simulink model "VCU_SW"  (R2020b)
settings: Solver=FixedStepDiscrete  StartTime=0.0  StopTime=inf  FixedStep=1e-2  RelTol=1e-3
PreLoadFcn:
  | RTWConfigurationCB('preloadfcn', bdroot);
InitFcn:
  | loadvar_ttc500
undefined symbols (not defined in the file or in its folder): BrkPedalTypes, CabMovModeTypes, cFuseTempSensAcc_X, cFuseTempSensAcc_Y, cFuseTempSensVal_X, cFuseTempSensVal_Y, cTMSTempSensVal_X, cTMSTempSensVal_Y, cTransferCaseSpeedRatio, diag_state, DoorsPositionTypes, dP_filter_Y, DriverOccClassSystemTypes, ErrorValueTypes, fatal_error_callback, IO_ADC_NO_RANGE, LadderStatusTypes, pAnalogCabRotSensAcc, pAnalogCabRotSensMaxVolt, pAnalogCabRotSensMinVolt, pAnalogCabRotSensRange, pAnalogCabRotSensZeroVolt, pBrkActivePress, pCabTiltSensAcc, pCabTiltSensMaxCur, pCabTiltSensMinCur, pDistanceCorrection, pECANManual_BPNEnable, pECANManual_BPNEnabler_Flag, pFilterSensAccRes, pHDirMaxDiffFrq, pHDirSensHighLvl, pHDirSensLowLvl, pMainGearRatio, pMaxFilterSensRes, pMaxFirstPedalSensValue, pMaxFuseTempSensRes, pMaxPressLoss, pMaxPressSensCurrent, pMaxPressValue, pMaxPressValueHydMotAndPump, pMaxPressValueParkDrain, pMaxSecondPedalSensValue, pMaxTempSensVoltage, pMaxTempValue, pMaxTMSTempSensRes, pMinFilterSensRes, pMinFirstPedalSensValue, pMinFuseTempSensRes, pMinPressLoss, pMinPressSensCurrent, pMinPressValue, pMinSecondPedalSensValue, pMinTempSensVoltage, pMinTempValue, pMinTMSTempSensRes, pMotorRingTeethNum, pPedalSensAccuracyPct, pPedalSensAccuracyVolt, pPressLossTreshhold ... (+20)
libraries: TTlibrary x271, canmsglib x128, simulink x88
(part 13 of 17)

== system VCU_SW/OutputLayer/OutputNetwork/OutputCCAN/SetCCAN1000msec/Eletcric_current_info ==
  CANPack_Electric_current_info : canmsglib/CAN Pack  MsgList=(none)  MsgName=Electric_current_info  MsgIDType=Extended (29-bit identifier)  MsgIdentifier=419386874  MsgLength=8  Remote=off  ApplyMinMax=off  BusOutput=on  SignalInfo={ 'equp_pump_cur', '48', '16', 'LE', 'unsigned', 'Standard', '0', '1', '0', '0', '65535'; 'front_drive_hydpump_cur', '0', '16', 'LE', 'unsigned', 'Standard', '0', '1', '0', '0', '65535'; 'hydmot_cur', '32', '16', 'LE', 'unsigned', 'Standard', '0', '1', '0', '0', '65535'; 'reverse_drive_hydpump_cur', '16', '16', 'LE', 'unsigned', 'Standard', '0', '1', '0', '0', '65535' }
      settings: SourceProductBaseCode=ME,XP,VN  DataFormat=manually specified signals
  Data Store Read : DataStoreRead  DataStoreName=OutputNetworkData  DataStoreElements=OutputNetworkData.CCAN.Electric_current_info.equp_pump_cur#OutputNetworkData.CCAN.Electric_current_info.front_drive_hydpump_cur#OutputNetworkData.CCAN.Electric_current_info.hydmot_cur#OutputNetworkData.CCAN.Electric_current_info.reverse_drive_hydpump_cur
  Terminator1 : Terminator
  transmit_message_electric_current_info : TTlibrary/CAN/transmit_message_name  channel=IO_CAN_CHANNEL_1  id_format=IO_CAN_STD_FRAME  retranslation=off  io_error=on  sample_time=-1
      settings: SourceProductName=TT control 500 series
  wires:
  transmit_message_electric_current_info/1 -> Terminator1/1  "error_tx_transmit_message_electric_current_info"
  CANPack_Electric_current_info/1 -> transmit_message_electric_current_info/1
  Data Store Read/1 -> CANPack_Electric_current_info/1
  Data Store Read/2 -> CANPack_Electric_current_info/2
  Data Store Read/3 -> CANPack_Electric_current_info/3
  Data Store Read/4 -> CANPack_Electric_current_info/4

== system VCU_SW/OutputLayer/OutputNetwork/OutputCCAN/SetCCAN1000msec/Eletcric_info ==
  CANPack_Electric_info : canmsglib/CAN Pack  MsgList=(none)  MsgName=Electric_info  MsgIDType=Extended (29-bit identifier)  MsgIdentifier=419387130  MsgLength=8  Remote=off  ApplyMinMax=off  BusOutput=on  SignalInfo={ 'bort_batt_voltage_lvl', '0', '8', 'LE', 'unsigned', 'Standard', '0', '1', '0', '0', '255'; 'can1_sts', '32', '2', 'LE', 'unsigned', 'Standard', '0', '1', '0', '0', '3'; 'can2_sts', '34', '2', 'LE', 'unsigned', 'Standard', '0', '1', '0', '0', '3'; 'can3_sts', '36', '2', 'LE', 'unsigned', 'Standard', '0', '1', '0', '0', '3'; 'can4_sts', '38', '2', 'LE', 'unsigned', 'Standard', '0', '1', '0', '0', '3'; 'can5_sts', '40', '2', 'LE', 'unsigned', 'Standard', '0', '1', '0', '0', '3'; 'can6_sts', '42', '2', 'LE', 'unsigned', 'Standard', '0', '1', '0', '0', '3'; 'lower_gen_signal', '10', '2', 'LE', 'unsigned', 'Standard', '0', '1', '0', '0', '3'; 'str_brk_pump_cur', '16', '16', 'LE', 'unsigned', 'Standard', '0', '1', '0', '0', '65535'; 'upper_gen_signal', '8', '2', 'LE', 'unsigned', 'Standard', '0', '1', '0', '0', '3' }
      settings: SourceProductBaseCode=ME,XP,VN  DataFormat=manually specified signals
  Data Store Read : DataStoreRead  DataStoreName=OutputNetworkData  DataStoreElements=OutputNetworkData.CCAN.Electric_info.bort_batt_voltage_lvl#OutputNetworkData.CCAN.Electric_info.can1_sts#OutputNetworkData.CCAN.Electric_info.can2_sts#OutputNetworkData.CCAN.Electric_info.can3_sts#OutputNetworkData.CCAN.Electric_info.can4_sts#OutputNetworkData.CCAN.Electric_info.can5_sts#OutputNetworkData.CCAN.Electric_info.can6_sts#OutputNetworkData.CCAN.Electric_info.lower_gen_signal#OutputNetworkData.CCAN.Electric_info.str_brk_pump_cur#OutputNetworkData.CCAN.Electric_info.bort_batt_voltage_lvl
  Terminator1 : Terminator
  transmit_message_electric_info : TTlibrary/CAN/transmit_message_name  channel=IO_CAN_CHANNEL_1  id_format=IO_CAN_STD_FRAME  retranslation=off  io_error=on  sample_time=-1
      settings: SourceProductName=TT control 500 series
  wires:
  CANPack_Electric_info/1 -> transmit_message_electric_info/1
  transmit_message_electric_info/1 -> Terminator1/1  "error_tx_transmit_message_electric_info"
  Data Store Read/1 -> CANPack_Electric_info/1
  Data Store Read/2 -> CANPack_Electric_info/2
  Data Store Read/3 -> CANPack_Electric_info/3
  Data Store Read/4 -> CANPack_Electric_info/4
  Data Store Read/5 -> CANPack_Electric_info/5
  Data Store Read/6 -> CANPack_Electric_info/6
  Data Store Read/7 -> CANPack_Electric_info/7
  Data Store Read/8 -> CANPack_Electric_info/8
  Data Store Read/9 -> CANPack_Electric_info/9
  Data Store Read/10 -> CANPack_Electric_info/10

== system VCU_SW/OutputLayer/OutputNetwork/OutputCCAN/SetCCAN1000msec/HTR ==
  CANPack_HTR : canmsglib/CAN Pack  MsgList=(none)  MsgName=HTR  MsgIDType=Extended (29-bit identifier)  MsgIdentifier=419327482  MsgLength=8  Remote=off  ApplyMinMax=off  BusOutput=on  SignalInfo={ 'AuxiliaryHeaterMode', '24', '4', 'LE', 'unsigned', 'Standard', '0', '1', '0', '0', '15' }
      settings: SourceProductBaseCode=ME,XP,VN  DataFormat=manually specified signals
  Data Store Read1 : DataStoreRead  DataStoreName=OutputNetworkData  DataStoreElements=OutputNetworkData.CCAN.HTR.AuxiliaryHeaterMode
  Terminator1 : Terminator
  transmit_message_htr : TTlibrary/CAN/transmit_message_name  channel=IO_CAN_CHANNEL_1  id_format=IO_CAN_STD_FRAME  retranslation=off  io_error=on  sample_time=-1
      settings: SourceProductName=TT control 500 series
  wires:
  CANPack_HTR/1 -> transmit_message_htr/1
  Data Store Read1/1 -> CANPack_HTR/1
  transmit_message_htr/1 -> Terminator1/1  "error_tx_transmit_message_htr"

== system VCU_SW/OutputLayer/OutputNetwork/OutputCCAN/SetCCAN1000msec/Hyd_transm_info ==
  CANPack_Hyd_transm_info : canmsglib/CAN Pack  MsgList=(none)  MsgName=Hyd_transm_info  MsgIDType=Extended (29-bit identifier)  MsgIdentifier=419386362  MsgLength=8  Remote=off  ApplyMinMax=off  BusOutput=on  SignalInfo={ 'front_drive_line_press', '0', '8', 'LE', 'unsigned', 'Standard', '0', '2', '0', '0', '510'; 'hyd_mot_temp_sens', '16', '8', 'LE', 'unsigned', 'Standard', '0', '1', '-40', '-40', '210'; 'hyd_pump_temp_sens', '24', '8', 'LE', 'unsigned', 'Standard', '0', '1', '-40', '-40', '210'; 'hydmot_direct_sens', '40', '2', 'LE', 'unsigned', 'Standard', '0', '1', '0', '0', '3'; 'hydpump_direct_sens', '48', '2', 'LE', 'unsigned', 'Standard', '0', '1', '0', '0', '3'; 'hydpump_washer_lean_sens', '32', '8', 'LE', 'unsigned', 'Standard', '0', '1', '0', '0', '255'; 'rear_drive_line_press', '8', '8', 'LE', 'unsigned', 'Standard', '0', '2', '0', '0', '510' }
      settings: SourceProductBaseCode=ME,XP,VN  DataFormat=manually specified signals
  Data Store Read : DataStoreRead  DataStoreName=OutputNetworkData  DataStoreElements=OutputNetworkData.CCAN.Hyd_transm_info.front_drive_line_press#OutputNetworkData.CCAN.Hyd_transm_info.hyd_mot_temp_sens#OutputNetworkData.CCAN.Hyd_transm_info.hyd_pump_temp_sens#OutputNetworkData.CCAN.Hyd_transm_info.hydmot_direct_sens#OutputNetworkData.CCAN.Hyd_transm_info.hydpump_direct_sens#OutputNetworkData.CCAN.Hyd_transm_info.hydpump_washer_lean_sens#OutputNetworkData.CCAN.Hyd_transm_info.rear_drive__line_press
  Terminator1 : Terminator
  transmit_message_hyd_transm_info : TTlibrary/CAN/transmit_message_name  channel=IO_CAN_CHANNEL_1  id_format=IO_CAN_STD_FRAME  retranslation=off  io_error=on  sample_time=-1
      settings: SourceProductName=TT control 500 series
  wires:
  transmit_message_hyd_transm_info/1 -> Terminator1/1  "error_tx_transmit_message_hyd_transm_info"
  CANPack_Hyd_transm_info/1 -> transmit_message_hyd_transm_info/1
  Data Store Read/1 -> CANPack_Hyd_transm_info/1
  Data Store Read/2 -> CANPack_Hyd_transm_info/2
  Data Store Read/3 -> CANPack_Hyd_transm_info/3
  Data Store Read/4 -> CANPack_Hyd_transm_info/4
  Data Store Read/5 -> CANPack_Hyd_transm_info/5
  Data Store Read/6 -> CANPack_Hyd_transm_info/6
  Data Store Read/7 -> CANPack_Hyd_transm_info/7

== system VCU_SW/OutputLayer/OutputNetwork/OutputCCAN/SetCCAN1000msec/Hyd_transm_speed_info ==
  CANPack_Hyd_transm_speed_info : canmsglib/CAN Pack  MsgList=(none)  MsgName=Hyd_transm_speed_info  MsgIDType=Extended (29-bit identifier)  MsgIdentifier=419386618  MsgLength=8  Remote=off  ApplyMinMax=off  BusOutput=on  SignalInfo={ 'hydmot_speed_sens_1', '32', '16', 'LE', 'unsigned', 'Standard', '0', '0.125', '0', '0', '8191.88'; 'hydmot_speed_sens_2', '48', '16', 'LE', 'unsigned', 'Standard', '0', '0.125', '0', '0', '8191.88'; 'hydpump_speed_sens_1', '0', '16', 'LE', 'unsigned', 'Standard', '0', '0.125', '0', '0', '8191.875'; 'hydpump_speed_sens_2', '16', '16', 'LE', 'unsigned', 'Standard', '0', '0.125', '0', '0', '8191.875' }
      settings: SourceProductBaseCode=ME,XP,VN  DataFormat=manually specified signals
  Data Store Read : DataStoreRead  DataStoreName=OutputNetworkData  DataStoreElements=OutputNetworkData.CCAN.Hyd_transm_speed_info.hydmot_speed_sens_1#OutputNetworkData.CCAN.Hyd_transm_speed_info.hydmot_speed_sens_2#OutputNetworkData.CCAN.Hyd_transm_speed_info.hydpump_speed_sens_1#OutputNetworkData.CCAN.Hyd_transm_speed_info.hydpump_speed_sens_2
  Data Type Conversion{,1..3} (4 alike) : DataTypeConversion  OutDataTypeStr=single
  Terminator1 : Terminator
  transmit_message_hyd_transm_speed_info : TTlibrary/CAN/transmit_message_name  channel=IO_CAN_CHANNEL_1  id_format=IO_CAN_STD_FRAME  retranslation=off  io_error=on  sample_time=-1
      settings: SourceProductName=TT control 500 series
  wires:
  CANPack_Hyd_transm_speed_info/1 -> transmit_message_hyd_transm_speed_info/1
  transmit_message_hyd_transm_speed_info/1 -> Terminator1/1  "error_tx_transmit_message_hyd_transm_speed_info"
  Data Store Read/1 -> Data Type Conversion/1
  Data Store Read/2 -> Data Type Conversion1/1
  Data Store Read/3 -> Data Type Conversion2/1
  Data Store Read/4 -> Data Type Conversion3/1
  Data Type Conversion/1 -> CANPack_Hyd_transm_speed_info/1
  Data Type Conversion1/1 -> CANPack_Hyd_transm_speed_info/2
  Data Type Conversion2/1 -> CANPack_Hyd_transm_speed_info/3
  Data Type Conversion3/1 -> CANPack_Hyd_transm_speed_info/4

== system VCU_SW/OutputLayer/OutputNetwork/OutputCCAN/SetCCAN1000msec/LCMD ==
  CANPack_LCMD_VCU : canmsglib/CAN Pack  MsgList=(none)  MsgName=LCMD_VCU  MsgIDType=Extended (29-bit identifier)  MsgIdentifier=217989626  MsgLength=3  Remote=off  ApplyMinMax=off  BusOutput=on  SignalInfo={ 'CenterStopLightCmd', '18', '2', 'LE', 'unsigned', 'Standard', '0', '1', '0', '0', '3'; 'LeftStopLightCmd', '22', '2', 'LE', 'unsigned', 'Standard', '0', '1', '0', '0', '3'; 'RightStopLightCmd', '20', '2', 'LE', 'unsigned', 'Standard', '0', '1', '0', '0', '3' }
      settings: SourceProductBaseCode=ME,XP,VN  DataFormat=manually specified signals
  Data Store Read1 : DataStoreRead  DataStoreName=OutputNetworkData  DataStoreElements=OutputNetworkData.CCAN.LD_out.CenterStopLight#OutputNetworkData.CCAN.LD_out.LeftStopLight#OutputNetworkData.CCAN.LD_out.RightStopLight
  Terminator1 : Terminator
  transmit_message_lcmd_vcu : TTlibrary/CAN/transmit_message_name  channel=IO_CAN_CHANNEL_1  id_format=IO_CAN_STD_FRAME  retranslation=off  io_error=on  sample_time=-1
      settings: SourceProductName=TT control 500 series
  wires:
  Data Store Read1/3 -> CANPack_LCMD_VCU/3
  Data Store Read1/2 -> CANPack_LCMD_VCU/2
  Data Store Read1/1 -> CANPack_LCMD_VCU/1
  transmit_message_lcmd_vcu/1 -> Terminator1/1  "error_tx_transmit_message_lcmd_vcu"
  CANPack_LCMD_VCU/1 -> transmit_message_lcmd_vcu/1

== system VCU_SW/OutputLayer/OutputNetwork/OutputCCAN/SetCCAN1000msec/MTUInformationArea ==
  CANPack_MTUInformationArea : canmsglib/CAN Pack  MsgList=(none)  MsgName=MTUInformationArea  MsgIDType=Extended (29-bit identifier)  MsgIdentifier=419386106  MsgLength=8  Remote=off  ApplyMinMax=off  BusOutput=on  SignalInfo={ 'info_area_id', '0', '8', 'LE', 'unsigned', 'Standard', '0', '1', '0', '0', '255' }
      settings: SourceProductBaseCode=ME,XP,VN  DataFormat=manually specified signals
  Ground : Ground
  Terminator1 : Terminator
  transmit_message_mtu_information_area : TTlibrary/CAN/transmit_message_name  channel=IO_CAN_CHANNEL_1  id_format=IO_CAN_STD_FRAME  retranslation=off  io_error=on  sample_time=-1
      settings: SourceProductName=TT control 500 series
  wires:
  CANPack_MTUInformationArea/1 -> transmit_message_mtu_information_area/1
  Ground/1 -> CANPack_MTUInformationArea/1
  transmit_message_mtu_information_area/1 -> Terminator1/1  "error_tx_transmit_message_mtu_information_area"

== system VCU_SW/OutputLayer/OutputNetwork/OutputCCAN/SetCCAN1000msec/TCI ==
  CANPack_TCI : canmsglib/CAN Pack  MsgList=(none)  MsgName=TCI  MsgIDType=Extended (29-bit identifier)  MsgIdentifier=419267578  MsgLength=8  Remote=off  ApplyMinMax=off  BusOutput=on  SignalInfo={ 'Transfer_Case_Status', '0', '3', 'LE', 'unsigned', 'Standard', '0', '1', '0', '0', '7' }
      settings: SourceProductBaseCode=ME,XP,VN  DataFormat=manually specified signals
  Data Store Read1 : DataStoreRead  DataStoreName=OutputNetworkData  DataStoreElements=OutputNetworkData.CCAN.TCI.Transfer_Case_Status
  Terminator1 : Terminator
  transmit_message_tci : TTlibrary/CAN/transmit_message_name  channel=IO_CAN_CHANNEL_1  id_format=IO_CAN_STD_FRAME  retranslation=off  io_error=on  sample_time=-1
      settings: SourceProductName=TT control 500 series
  wires:
  transmit_message_tci/1 -> Terminator1/1  "error_tx_transmit_message_tci"
  Data Store Read1/1 -> CANPack_TCI/1
  CANPack_TCI/1 -> transmit_message_tci/1

== system VCU_SW/OutputLayer/OutputNetwork/OutputCCAN/SetCCAN1000msec/TRF2 ==
  CANPack_TRF2 : canmsglib/CAN Pack  MsgList=(none)  MsgName=TRF2  MsgIDType=Extended (29-bit identifier)  MsgIdentifier=419272186  MsgLength=8  Remote=off  ApplyMinMax=off  BusOutput=on  SignalInfo={ 'Transmission_Overheat_Indicator', '4', '2', 'LE', 'unsigned', 'Standard', '0', '1', '0', '0', '3' }
      settings: SourceProductBaseCode=ME,XP,VN  DataFormat=manually specified signals
  Data Store Read1 : DataStoreRead  DataStoreName=OutputNetworkData  DataStoreElements=OutputNetworkData.CCAN.TRF2.Transmission_Overheat_Indicator
  Terminator1 : Terminator
  transmit_message_trf2 : TTlibrary/CAN/transmit_message_name  channel=IO_CAN_CHANNEL_1  id_format=IO_CAN_STD_FRAME  retranslation=off  io_error=on  sample_time=-1
      settings: SourceProductName=TT control 500 series
  wires:
  CANPack_TRF2/1 -> transmit_message_trf2/1
  Data Store Read1/1 -> CANPack_TRF2/1
  transmit_message_trf2/1 -> Terminator1/1  "error_tx_transmit_message_trf2"

== system VCU_SW/OutputLayer/OutputNetwork/OutputCCAN/SetCCAN1000msec/VH ==
  CANPack_VH : canmsglib/CAN Pack  MsgList=(none)  MsgName=VH  MsgIDType=Extended (29-bit identifier)  MsgIdentifier=419358714  MsgLength=8  Remote=off  ApplyMinMax=off  BusOutput=on  SignalInfo={ 'TotalVehicleHours', '0', '32', 'LE', 'unsigned', 'Standard', '0', '0.05', '0', '0', '210554060.75'; 'TripVehicleHours', '32', '32', 'LE', 'unsigned', 'Standard', '0', '0.05', '0', '0', '210554000' }
      settings: SourceProductBaseCode=ME,XP,VN  DataFormat=manually specified signals
  Data Store Read1 : DataStoreRead  DataStoreName=OutputNetworkData  DataStoreElements=OutputNetworkData.CCAN.VH.TotalVehicleHours
  Data Store Read2 : DataStoreRead  DataStoreName=OutputNetworkData  DataStoreElements=OutputNetworkData.CCAN.VH.TripVehicleHours
  Terminator1 : Terminator
  transmit_message_vh : TTlibrary/CAN/transmit_message_name  channel=IO_CAN_CHANNEL_1  id_format=IO_CAN_STD_FRAME  retranslation=off  io_error=on  sample_time=-1
      settings: SourceProductName=TT control 500 series
  wires:
  CANPack_VH/1 -> transmit_message_vh/1
  Data Store Read1/1 -> CANPack_VH/1
  transmit_message_vh/1 -> Terminator1/1  "error_tx_transmit_message_vh"
  Data Store Read2/1 -> CANPack_VH/2

== system VCU_SW/OutputLayer/OutputNetwork/OutputCCAN/SetCCAN100msec/CCVS1 ==
  CANPack_CCVS1 : canmsglib/CAN Pack  MsgList=(none)  MsgName=CCVS1  MsgIDType=Extended (29-bit identifier)  MsgIdentifier=419361274  MsgLength=8  Remote=off  ApplyMinMax=off  BusOutput=on  SignalInfo={ 'Brake_Switch', '28', '2', 'LE', 'unsigned', 'Standard', '0', '1', '0', '0', '3'; 'PTO_Governor_State', '48', '5', 'LE', 'unsigned', 'Standard', '0', '1', '0', '0', '32'; 'Parking_Brake_Switch', '2', '2', 'LE', 'unsigned', 'Standard', '0', '1', '0', '0', '3'; 'Wheel_Based_Vehicle_Speed', '8', '16', 'LE', 'unsigned', 'Standard', '0', '0.0039', '0', '0', '250' }
      settings: SourceProductBaseCode=ME,XP,VN  DataFormat=manually specified signals
  Data Store Read1 : DataStoreRead  DataStoreName=OutputNetworkData  DataStoreElements=OutputNetworkData.CCAN.CCVS1.Brake_Switch#OutputNetworkData.CCAN.CCVS1.PTO_Governor_State#OutputNetworkData.CCAN.CCVS1.Parking_Brake_Switch#OutputNetworkData.CCAN.CCVS1.Wheel_Based_Vehicle_Speed
  Terminator1 : Terminator
  transmit_message_ccvs1 : TTlibrary/CAN/transmit_message_name  channel=IO_CAN_CHANNEL_1  id_format=IO_CAN_STD_FRAME  retranslation=off  io_error=on  sample_time=-1
      settings: SourceProductName=TT control 500 series
  wires:
  Data Store Read1/2 -> CANPack_CCVS1/2
  Data Store Read1/3 -> CANPack_CCVS1/3
  Data Store Read1/4 -> CANPack_CCVS1/4
  transmit_message_ccvs1/1 -> Terminator1/1  "error_tx_transmit_message_ccvs1"
  Data Store Read1/1 -> CANPack_CCVS1/1
  CANPack_CCVS1/1 -> transmit_message_ccvs1/1

== system VCU_SW/OutputLayer/OutputNetwork/OutputCCAN/SetCCAN100msec/Cabine Angles ==
  CANPack_CabineAngles : canmsglib/CAN Pack  MsgList=(none)  MsgName=CabineAngles  MsgIDType=Extended (29-bit identifier)  MsgIdentifier=419374330  MsgLength=8  Remote=off  ApplyMinMax=off  BusOutput=on  SignalInfo={ 'CabineLateralAngle', '0', '8', 'LE', 'unsigned', 'Standard', '0', '0.4', '-50', '-50', '50'; 'CabineRotationAngle', '16', '8', 'LE', 'unsigned', 'Standard', '0', '0.5', '-120', '-120', '120'; 'CabineTraverseAngle', '8', '8', 'LE', 'unsigned', 'Standard', '0', '0.4', '-50', '-50', '50'; 'FrameLateralAngle', '24', '8', 'LE', 'unsigned', 'Standard', '0', '0.4', '-50', '-50', '50'; 'FrameTraverselAngle', '32', '8', 'LE', 'unsigned', 'Standard', '0', '0.4', '-50', '-50', '50' }
      settings: SourceProductBaseCode=ME,XP,VN  DataFormat=manually specified signals
  Data Store Read1 : DataStoreRead  DataStoreName=OutputNetworkData  DataStoreElements=OutputNetworkData.CCAN.CabineAngles.CabineLateralAngle#OutputNetworkData.CCAN.CabineAngles.CabineRotationAngle#OutputNetworkData.CCAN.CabineAngles.CabineTraverseAngle#OutputNetworkData.CCAN.CabineAngles.FrameLateralAngle#OutputNetworkData.CCAN.CabineAngles.FrameTraverselAngle
  Terminator1 : Terminator
  transmit_message_cabine_angles : TTlibrary/CAN/transmit_message_name  channel=IO_CAN_CHANNEL_1  id_format=IO_CAN_STD_FRAME  retranslation=off  io_error=on  sample_time=-1
      settings: SourceProductName=TT control 500 series
  wires:
  Data Store Read1/5 -> CANPack_CabineAngles/5
  Data Store Read1/4 -> CANPack_CabineAngles/4
  Data Store Read1/3 -> CANPack_CabineAngles/3
  Data Store Read1/2 -> CANPack_CabineAngles/2
  transmit_message_cabine_angles/1 -> Terminator1/1  "error_tx_transmit_message_cabine_angles"
  Data Store Read1/1 -> CANPack_CabineAngles/1
  CANPack_CabineAngles/1 -> transmit_message_cabine_angles/1

== system VCU_SW/OutputLayer/OutputNetwork/OutputCCAN/SetCCAN100msec/Cabine Status  ==
  CANPack_CabineStatus : canmsglib/CAN Pack  MsgList=(none)  MsgName=CabineStatus  MsgIDType=Extended (29-bit identifier)  MsgIdentifier=419374074  MsgLength=8  Remote=off  ApplyMinMax=off  BusOutput=on  SignalInfo={ 'BackwardCabLean_Sts', '0', '2', 'LE', 'unsigned', 'Standard', '0', '1', '0', '0', '3'; 'CabRestoreDefaultRot_Sts', '8', '2', 'LE', 'unsigned', 'Standard', '0', '1', '0', '0', '3'; 'CabRestoreDefaultTilt_Sts', '10', '2', 'LE', 'unsigned', 'Standard', '0', '1', '0', '0', '3'; 'CabStabilization_Sts', '12', '2', 'LE', 'unsigned', 'Standard', '0', '1', '0', '0', '3'; 'ForwardCabLean_Sts', '2', '2', 'LE', 'unsigned', 'Standard', '0', '1', '0', '0', '3'; 'LeftCabLean_Sts', '4', '2', 'LE', 'unsigned', 'Standard', '0', '1', '0', '0', '3'; 'RightCabLean_Sts', '6', '2', 'LE', 'unsigned', 'Standard', '0', '1', '0', '0', '3' }
      settings: SourceProductBaseCode=ME,XP,VN  DataFormat=manually specified signals
  Data Store Read1 : DataStoreRead  DataStoreName=OutputNetworkData  DataStoreElements=OutputNetworkData.CCAN.CabineStatus.BackwardCabLean_Sts#OutputNetworkData.CCAN.CabineStatus.CabRestoreDefaultRot_Sts#OutputNetworkData.CCAN.CabineStatus.CabRestoreDefaultTilt_Sts#OutputNetworkData.CCAN.CabineStatus.CabStabilization_Sts#OutputNetworkData.CCAN.CabineStatus.ForwardCabLean_Sts#OutputNetworkData.CCAN.CabineStatus.LeftCabLean_Sts#OutputNetworkData.CCAN.CabineStatus.RightCabLean_Sts
  Terminator1 : Terminator
  transmit_message_cabine_status : TTlibrary/CAN/transmit_message_name  channel=IO_CAN_CHANNEL_1  id_format=IO_CAN_STD_FRAME  retranslation=off  io_error=on  sample_time=-1
      settings: SourceProductName=TT control 500 series
  wires:
  Data Store Read1/7 -> CANPack_CabineStatus/7
  Data Store Read1/6 -> CANPack_CabineStatus/6
  Data Store Read1/5 -> CANPack_CabineStatus/5
  Data Store Read1/4 -> CANPack_CabineStatus/4
  Data Store Read1/3 -> CANPack_CabineStatus/3
  Data Store Read1/2 -> CANPack_CabineStatus/2
  transmit_message_cabine_status/1 -> Terminator1/1  "error_tx_transmit_message_cabine_status"
  Data Store Read1/1 -> CANPack_CabineStatus/1
  CANPack_CabineStatus/1 -> transmit_message_cabine_status/1

== system VCU_SW/OutputLayer/OutputNetwork/OutputCCAN/SetCCAN100msec/EBC1 ==
  CANPack_EBC1 : canmsglib/CAN Pack  MsgList=(none)  MsgName=EBC1  MsgIDType=Extended (29-bit identifier)  MsgIdentifier=418382330  MsgLength=8  Remote=off  ApplyMinMax=off  BusOutput=on  SignalInfo={ 'ABS_EBS_Amber_Warning_Signal', '44', '2', 'LE', 'unsigned', 'Standard', '0', '1', '0', '0', '3'; 'EBS_Red_Warning_Signal', '42', '2', 'LE', 'unsigned', 'Standard', '0', '1', '0', '0', '3' }
      settings: SourceProductBaseCode=ME,XP,VN  DataFormat=manually specified signals
  Data Store Read1 : DataStoreRead  DataStoreName=OutputNetworkData  DataStoreElements=OutputNetworkData.CCAN.EBC1.ABS_EBS_Amber_Warning_Signal#OutputNetworkData.CCAN.EBC1.EBS_Red_Warning_Signal
  Terminator1 : Terminator
  transmit_message_ebc1 : TTlibrary/CAN/transmit_message_name  channel=IO_CAN_CHANNEL_1  id_format=IO_CAN_STD_FRAME  retranslation=off  io_error=on  sample_time=-1
      settings: SourceProductName=TT control 500 series
  wires:
  Data Store Read1/2 -> CANPack_EBC1/2
  transmit_message_ebc1/1 -> Terminator1/1  "error_tx_transmit_message_ebc1"
  Data Store Read1/1 -> CANPack_EBC1/1
  CANPack_EBC1/1 -> transmit_message_ebc1/1

== system VCU_SW/OutputLayer/OutputNetwork/OutputCCAN/SetCCAN100msec/ETC2 ==
  CANPack_ETC2 : canmsglib/CAN Pack  MsgList=(none)  MsgName=ETC2  MsgIDType=Extended (29-bit identifier)  MsgIdentifier=418383354  MsgLength=8  Remote=off  ApplyMinMax=off  BusOutput=on  SignalInfo={ 'Transmission_Actual_Gear_Ratio', '8', '16', 'LE', 'unsigned', 'Standard', '0', '0.001', '0', '0', '64.255'; 'Transmission_Current_Gear', '24', '8', 'LE', 'unsigned', 'Standard', '0', '1', '0', '0', '255'; 'Transmission_Current_Range', '48', '16', 'LE', 'unsigned', 'Standard', '0', '1', '0', '0', '65535'; 'Transmission_Requested_Range', '32', '16', 'LE', 'unsigned', 'Standard', '0', '1', '0', '0', '65535'; 'Transmission_Selected_Gear', '0', '8', 'LE', 'unsigned', 'Standard', '0', '1', '0', '0', '255' }
      settings: SourceProductBaseCode=ME,XP,VN  DataFormat=manually specified signals
  Data Store Read : DataStoreRead  DataStoreName=OutputNetworkData  DataStoreElements=OutputNetworkData.CCAN.ETC2.Transmission_Actual_Gear_Ratio#OutputNetworkData.CCAN.ETC2.Transmission_Current_Gear#OutputNetworkData.CCAN.ETC2.Transmission_Current_Range#OutputNetworkData.CCAN.ETC2.Transmission_Requested_Range#OutputNetworkData.CCAN.ETC2.Transmission_Selected_Gear
  Terminator : Terminator
  transmit_message_etc2 : TTlibrary/CAN/transmit_message_name  channel=IO_CAN_CHANNEL_1  id_format=IO_CAN_STD_FRAME  retranslation=off  io_error=on  sample_time=-1
      settings: SourceProductName=TT control 500 series
  wires:
  Data Store Read/5 -> CANPack_ETC2/5
  Data Store Read/4 -> CANPack_ETC2/4
  Data Store Read/3 -> CANPack_ETC2/3
  Data Store Read/2 -> CANPack_ETC2/2
  Data Store Read/1 -> CANPack_ETC2/1
  CANPack_ETC2/1 -> transmit_message_etc2/1
  transmit_message_etc2/1 -> Terminator/1  "error_tx_transmit_message_etc2"

== system VCU_SW/OutputLayer/OutputNetwork/OutputCCAN/SetCCAN100msec/ETC7 ==
  CANPack_ETC7 : canmsglib/CAN Pack  MsgList=(none)  MsgName=ETC7  MsgIDType=Extended (29-bit identifier)  MsgIdentifier=419318522  MsgLength=8  Remote=off  ApplyMinMax=off  BusOutput=on  SignalInfo={ 'Trans_Mode_1_Ind', '22', '2', 'LE', 'unsigned', 'Standard', '0', '1', '0', '0', '3'; 'Trans_Mode_2_Ind', '20', '2', 'LE', 'unsigned', 'Standard', '0', '1', '0', '0', '3'; 'Transmission_Service_Indicator', '2', '2', 'LE', 'unsigned', 'Standard', '0', '1', '0', '0', '3'; 'Transmission_Shift_Inhibit_Ind', '14', '2', 'LE', 'unsigned', 'Standard', '0', '1', '0', '0', '3'; 'Transmission_Warning_Indicator', '42', '2', 'LE', 'unsigned', 'Standard', '0', '1', '0', '0', '3' }
      settings: SourceProductBaseCode=ME,XP,VN  DataFormat=manually specified signals
  Data Store Read1 : DataStoreRead  DataStoreName=OutputNetworkData  DataStoreElements=OutputNetworkData.CCAN.ETC7.Trans_Mode_1_Ind#OutputNetworkData.CCAN.ETC7.Trans_Mode_2_Ind#OutputNetworkData.CCAN.ETC7.Transmission_Service_Indicator#OutputNetworkData.CCAN.ETC7.Transmission_Shift_Inhibit_Ind#OutputNetworkData.CCAN.ETC7.Transmission_Warning_Indicator
  Terminator1 : Terminator
  transmit_message_etc7 : TTlibrary/CAN/transmit_message_name  channel=IO_CAN_CHANNEL_1  id_format=IO_CAN_STD_FRAME  retranslation=off  io_error=on  sample_time=-1
      settings: SourceProductName=TT control 500 series
  wires:
  Data Store Read1/5 -> CANPack_ETC7/5
  Data Store Read1/4 -> CANPack_ETC7/4
  Data Store Read1/3 -> CANPack_ETC7/3
  Data Store Read1/2 -> CANPack_ETC7/2
  transmit_message_etc7/1 -> Terminator1/1  "error_tx_transmit_message_etc7"
  Data Store Read1/1 -> CANPack_ETC7/1
  CANPack_ETC7/1 -> transmit_message_etc7/1

== system VCU_SW/OutputLayer/OutputNetwork/OutputCCAN/SetCCAN100msec/Fuel Filter Heater Status  ==
  CANPack_FuelFilterHeaterStatus : canmsglib/CAN Pack  MsgList=(none)  MsgName=FuelFilterHeaterStatus  MsgIDType=Extended (29-bit identifier)  MsgIdentifier=419374586  MsgLength=8  Remote=off  ApplyMinMax=off  BusOutput=on  SignalInfo={ 'FuelCoarseFilterHeatingStt', '0', '2', 'LE', 'unsigned', 'Standard', '0', '1', '0', '0', '3' }
      settings: SourceProductBaseCode=ME,XP,VN  DataFormat=manually specified signals
  Data Store Read1 : DataStoreRead  DataStoreName=OutputNetworkData  DataStoreElements=OutputNetworkData.CCAN.FuelFilterHeaterStatus.FuelCoarseFilterHeatingStt
  Terminator1 : Terminator
  transmit_message_fuel_filter_heater_status : TTlibrary/CAN/transmit_message_name  channel=IO_CAN_CHANNEL_1  id_format=IO_CAN_STD_FRAME  retranslation=off  io_error=on  sample_time=-1
      settings: SourceProductName=TT control 500 series
  wires:
  transmit_message_fuel_filter_heater_status/1 -> Terminator1/1  "error_tx_transmit_message_fuel_filter_heater_status"
  Data Store Read1/1 -> CANPack_FuelFilterHeaterStatus/1
  CANPack_FuelFilterHeaterStatus/1 -> transmit_message_fuel_filter_heater_status/1

== system VCU_SW/OutputLayer/OutputNetwork/OutputCCAN/SetCCAN100msec/FuelUsingOEM ==
  CANPack_FuelUsingOEM : canmsglib/CAN Pack  MsgList=(none)  MsgName=FuelUsingOEM  MsgIDType=Extended (29-bit identifier)  MsgIdentifier=419385850  MsgLength=8  Remote=off  ApplyMinMax=off  BusOutput=on  SignalInfo={ 'moment_fuel_rate_l_h', '32', '16', 'LE', 'unsigned', 'Standard', '0', '0.1', '0', '0', '6553.5'; 'moment_fuel_rate_l_km', '0', '16', 'LE', 'unsigned', 'Standard', '0', '0.1', '0', '0', '6553.5'; 'total_fuel_rate_l_h', '48', '16', 'LE', 'unsigned', 'Standard', '0', '0.1', '0', '0', '6553.5'; 'total_fuel_rate_l_km', '16', '16', 'LE', 'unsigned', 'Standard', '0', '0.1', '0', '0', '6553.5' }
      settings: SourceProductBaseCode=ME,XP,VN  DataFormat=manually specified signals
  Ground{,1..3} (4 alike) : Ground
  Terminator1 : Terminator
  transmit_message_fuel_using_oem : TTlibrary/CAN/transmit_message_name  channel=IO_CAN_CHANNEL_1  id_format=IO_CAN_STD_FRAME  retranslation=off  io_error=on  sample_time=-1
      settings: SourceProductName=TT control 500 series
  wires:
  CANPack_FuelUsingOEM/1 -> transmit_message_fuel_using_oem/1
  transmit_message_fuel_using_oem/1 -> Terminator1/1  "error_tx_transmit_message_fuel_using_oem"
  Ground/1 -> CANPack_FuelUsingOEM/1
  Ground1/1 -> CANPack_FuelUsingOEM/2
  Ground2/1 -> CANPack_FuelUsingOEM/3
  Ground3/1 -> CANPack_FuelUsingOEM/4

== system VCU_SW/OutputLayer/OutputNetwork/OutputCCAN/SetCCAN100msec/VD ==
  CANPack_VD : canmsglib/CAN Pack  MsgList=(none)  MsgName=VD  MsgIDType=Extended (29-bit identifier)  MsgIdentifier=419356922  MsgLength=8  Remote=off  ApplyMinMax=off  BusOutput=on  SignalInfo={ 'Total_Vehicle_Distance', '32', '32', 'LE', 'unsigned', 'Standard', '0', '0.125', '0', '0', '526385151.9'; 'Trip_Distance', '0', '32', 'LE', 'unsigned', 'Standard', '0', '0.125', '0', '0', '526385151.9' }
      settings: SourceProductBaseCode=ME,XP,VN  DataFormat=manually specified signals
  Data Store Read1 : DataStoreRead  DataStoreName=OutputNetworkData  DataStoreElements=OutputNetworkData.CCAN.VD.Total_Vehicle_Distance#OutputNetworkData.CCAN.VD.Trip_Distance
  Terminator1 : Terminator
  transmit_message_vd : TTlibrary/CAN/transmit_message_name  channel=IO_CAN_CHANNEL_1  id_format=IO_CAN_STD_FRAME  retranslation=off  io_error=on  sample_time=-1
      settings: SourceProductName=TT control 500 series
  wires:
  Data Store Read1/2 -> CANPack_VD/2
  CANPack_VD/1 -> transmit_message_vd/1
  Data Store Read1/1 -> CANPack_VD/1
  transmit_message_vd/1 -> Terminator1/1  "error_tx_transmit_message_vd"

== system VCU_SW/OutputLayer/OutputNetwork/OutputCCAN/SetCCAN100msec/VLVCMD_ MANIP_TABLE  ==
  CANPack_VLVCMD_MANIP_TABLE : canmsglib/CAN Pack  MsgList=(none)  MsgName=VLVCMD_MANIP_TABLE  MsgIDType=Extended (29-bit identifier)  MsgIdentifier=217985530  MsgLength=8  Remote=off  ApplyMinMax=off  BusOutput=on  SignalInfo={ 'FailSafeModeCmdManip', '22', '2', 'LE', 'unsigned', 'Standard', '0', '1', '0', '0', '3'; 'PortFlowCmdManip', '0', '8', 'LE', 'unsigned', 'Standard', '0', '1', '0', '0', '100'; 'ValveStateManip', '16', '4', 'LE', 'unsigned', 'Standard', '0', '1', '0', '0', '15' }
      settings: SourceProductBaseCode=ME,XP,VN  DataFormat=manually specified signals
  Data Store Read1 : DataStoreRead  DataStoreName=OutputNetworkData  DataStoreElements=OutputNetworkData.CCAN.VLVCMD_MANIP.FailSafeModeCmdManip#OutputNetworkData.CCAN.VLVCMD_MANIP.PortFlowCmdManip#OutputNetworkData.CCAN.VLVCMD_MANIP.ValveStateManip
  Terminator1 : Terminator
  transmit_message_vlvcmd_manip_table : TTlibrary/CAN/transmit_message_name  channel=IO_CAN_CHANNEL_1  id_format=IO_CAN_STD_FRAME  retranslation=off  io_error=on  sample_time=-1
      settings: SourceProductName=TT control 500 series
  wires:
  Data Store Read1/2 -> CANPack_VLVCMD_MANIP_TABLE/2
  Data Store Read1/3 -> CANPack_VLVCMD_MANIP_TABLE/3
  transmit_message_vlvcmd_manip_table/1 -> Terminator1/1  "error_tx_transmit_message_vlvcmd_manip_table"
  Data Store Read1/1 -> CANPack_VLVCMD_MANIP_TABLE/1
  CANPack_VLVCMD_MANIP_TABLE/1 -> transmit_message_vlvcmd_manip_table/1

== system VCU_SW/OutputLayer/OutputNetwork/OutputCCAN/SetCCAN500msec/Brake_circuits_manip_press ==
  CANPack_Brake_circuits_manip_press : canmsglib/CAN Pack  MsgList=(none)  MsgName=Brake_circuits_manip_press  MsgIDType=Extended (29-bit identifier)  MsgIdentifier=419385383  MsgLength=8  Remote=off  ApplyMinMax=off  BusOutput=on  SignalInfo={ 'front_ha_brake_pressure', '0', '8', 'LE', 'unsigned', 'Standard', '0', '1', '0', '0', '255'; 'front_work_brake_pressure', '24', '8', 'LE', 'unsigned', 'Standard', '0', '1', '0', '0', '255'; 'ls_hydpump_str_brk_pressure', '40', '8', 'LE', 'unsigned', 'Standard', '0', '1', '0', '0', '255'; 'manipulator_pressure', '56', '8', 'LE', 'unsigned', 'Standard', '0', '1', '0', '0', '255'; 'park_ha_brake_pressure', '16', '8', 'LE', 'unsigned', 'Standard', '0', '1', '0', '0', '255'; 'park_work_brake_pressure', '48', '8', 'LE', 'unsigned', 'Standard', '0', '1', '0', '0', '255'; 'rear_ha_brake_pressure', '8', '8', 'LE', 'unsigned', 'Standard', '0', '1', '0', '0', '255'; 'rear_work_brake_pressure', '32', '8', 'LE', 'unsigned', 'Standard', '0', '1', '0', '0', '255' }
      settings: SourceProductBaseCode=ME,XP,VN  DataFormat=manually specified signals
  Data Store Read : DataStoreRead  DataStoreName=OutputNetworkData  DataStoreElements=OutputNetworkData.CCAN.Brake_circuits_manip_press.front_ha_brake_pressure#OutputNetworkData.CCAN.Brake_circuits_manip_press.front_work_brake_pressure#OutputNetworkData.CCAN.Brake_circuits_manip_press.ls_hydpump_str_brk_pressure#OutputNetworkData.CCAN.Brake_circuits_manip_press.manipulator_pressure#OutputNetworkData.CCAN.Brake_circuits_manip_press.park_ha_brake_pressure#OutputNetworkData.CCAN.Brake_circuits_manip_press.park_work_brake_pressure#OutputNetworkData.CCAN.Brake_circuits_manip_press.rear_ha_brake_pressure#OutputNetworkData.CCAN.Brake_circuits_manip_press.rear_work_brake_pressure
  Terminator1 : Terminator
  transmit_message_brake_circuits_manip_press : TTlibrary/CAN/transmit_message_name  channel=IO_CAN_CHANNEL_1  id_format=IO_CAN_STD_FRAME  retranslation=off  io_error=on  sample_time=-1
      settings: SourceProductName=TT control 500 series
  wires:
  transmit_message_brake_circuits_manip_press/1 -> Terminator1/1  "error_tx_transmit_message_brake_circuits_manip_press"
  CANPack_Brake_circuits_manip_press/1 -> transmit_message_brake_circuits_manip_press/1
  Data Store Read/1 -> CANPack_Brake_circuits_manip_press/1
  Data Store Read/2 -> CANPack_Brake_circuits_manip_press/2
  Data Store Read/3 -> CANPack_Brake_circuits_manip_press/3
  Data Store Read/4 -> CANPack_Brake_circuits_manip_press/4
  Data Store Read/5 -> CANPack_Brake_circuits_manip_press/5
  Data Store Read/6 -> CANPack_Brake_circuits_manip_press/6
  Data Store Read/7 -> CANPack_Brake_circuits_manip_press/7
  Data Store Read/8 -> CANPack_Brake_circuits_manip_press/8

== system VCU_SW/OutputLayer/OutputNetwork/OutputCCAN/SetCCAN500msec/EAC1 ==
  CANPack_EAC1 : canmsglib/CAN Pack  MsgList=(none)  MsgName=EAC1  MsgIDType=Extended (29-bit identifier)  MsgIdentifier=418383354  MsgLength=8  Remote=off  ApplyMinMax=off  BusOutput=on  SignalInfo={ 'Diff_LockState_CenReal', '28', '2', 'LE', 'unsigned', 'Standard', '0', '1', '0', '0', '3'; 'Differential_LockState_CenFront', '26', '2', 'LE', 'unsigned', 'Standard', '0', '1', '0', '0', '3'; 'Differential_LockState_Central', '24', '2', 'LE', 'unsigned', 'Standard', '0', '1', '0', '0', '3' }
      settings: SourceProductBaseCode=ME,XP,VN  DataFormat=manually specified signals
  Data Store Read1 : DataStoreRead  DataStoreName=OutputNetworkData  DataStoreElements=OutputNetworkData.CCAN.EAC1_out.Diff_LockState_CenRear#OutputNetworkData.CCAN.EAC1_out.Differential_LockState_CenFront#OutputNetworkData.CCAN.EAC1_out.Differential_LockState_Central
  Terminator1 : Terminator
  transmit_message_eac1 : TTlibrary/CAN/transmit_message_name  channel=IO_CAN_CHANNEL_1  id_format=IO_CAN_STD_FRAME  retranslation=off  io_error=on  sample_time=-1
      settings: SourceProductName=TT control 500 series
  wires:
  Data Store Read1/3 -> CANPack_EAC1/3
  Data Store Read1/2 -> CANPack_EAC1/2
  CANPack_EAC1/1 -> transmit_message_eac1/1
  transmit_message_eac1/1 -> Terminator1/1  "error_tx_transmit_message_eac1"
  Data Store Read1/1 -> CANPack_EAC1/1

== system VCU_SW/OutputLayer/OutputNetwork/OutputCCAN/SetCCAN500msec/EFL//P1  ==
  CANPack_EFL_P1 : canmsglib/CAN Pack  MsgList=(none)  MsgName=EFL_P1  MsgIDType=Extended (29-bit identifier)  MsgIdentifier=419360762  MsgLength=8  Remote=off  ApplyMinMax=off  BusOutput=on  SignalInfo={ 'Engine_Coolant_Level', '56', '8', 'LE', 'unsigned', 'Standard', '0', '0.4', '0', '0', '100'; 'Engine_Oil_Pressure', '24', '8', 'LE', 'unsigned', 'Standard', '0', '4', '0', '0', '1000' }
      settings: SourceProductBaseCode=ME,XP,VN  DataFormat=manually specified signals
  Data Store Read1 : DataStoreRead  DataStoreName=OutputNetworkData  DataStoreElements=OutputNetworkData.CCAN.EFL_P1.Engine_Coolant_Level#OutputNetworkData.CCAN.EFL_P1.Engine_Oil_Pressure
  Terminator1 : Terminator
  transmit_message_efl_p1 : TTlibrary/CAN/transmit_message_name  channel=IO_CAN_CHANNEL_1  id_format=IO_CAN_STD_FRAME  retranslation=off  io_error=on  sample_time=-1
      settings: SourceProductName=TT control 500 series
  wires:
  Data Store Read1/2 -> CANPack_EFL_P1/2
  CANPack_EFL_P1/1 -> transmit_message_efl_p1/1
  transmit_message_efl_p1/1 -> Terminator1/1  "error_tx_transmit_message_efl_p1"
  Data Store Read1/1 -> CANPack_EFL_P1/1

== system VCU_SW/OutputLayer/OutputNetwork/OutputCCAN/SetCCAN500msec/EFL//P12 ==
  CANPack_DCDC_IN_Control1 : canmsglib/CAN Pack  MsgList=(none)  MsgName=EFL_P12  MsgIDType=Extended (29-bit identifier)  MsgIdentifier=419225594  MsgLength=8  Remote=off  ApplyMinMax=off  BusOutput=on  SignalInfo={ 'EngFuelFilterEstUseLife', '24', '8', 'LE', 'unsigned', 'Standard', '0', '1', '0', '0', '250' }
      settings: SourceProductBaseCode=ME,XP,VN  DataFormat=manually specified signals
  Data Store Read1 : DataStoreRead  DataStoreName=OutputNetworkData  DataStoreElements=OutputNetworkData.CCAN.EFL_P12.EngFuelFilterEstUseLife
  Terminator1 : Terminator
  transmit_message_dcdc_in_control1 : TTlibrary/CAN/transmit_message_name  channel=IO_CAN_CHANNEL_1  id_format=IO_CAN_STD_FRAME  retranslation=off  io_error=on  sample_time=-1
      settings: SourceProductName=TT control 500 series
  wires:
  CANPack_DCDC_IN_Control1/1 -> transmit_message_dcdc_in_control1/1
  transmit_message_dcdc_in_control1/1 -> Terminator1/1  "error_tx_transmit_message_dcdc_in_control1"
  Data Store Read1/1 -> CANPack_DCDC_IN_Control1/1

== system VCU_SW/OutputLayer/OutputNetwork/OutputCCAN/SetCCAN50msec/EEC1 ==
  CANPack_EEC1 : canmsglib/CAN Pack  MsgList=(none)  MsgName=EEC1  MsgIDType=Extended (29-bit identifier)  MsgIdentifier=418383098  MsgLength=8  Remote=off  ApplyMinMax=off  BusOutput=on  SignalInfo={ 'ActEngPercentTrq', '16', '8', 'LE', 'unsigned', 'Standard', '0', '1', '-125', '-125', '125'; 'ActEngPercentTrqHR', '4', '4', 'LE', 'unsigned', 'Standard', '0', '0.125', '0', '0', '0.875'; 'DrvrsDemandEngPercTrq', '8', '8', 'LE', 'unsigned', 'Standard', '0', '1', '-125', '-125', '125'; 'EngDemantPercTrq', '56', '8', 'LE', 'unsigned', 'Standard', '0', '1', '-125', '-125', '125'; 'EngStarterMode', '48', '4', 'LE', 'unsigned', 'Standard', '0', '1', '0', '0', '15'; 'EngTorqMode', '0', '4', 'LE', 'unsigned', 'Standard', '0', '1', '0', '0', '15'; 'EngineSpeed', '24', '16', 'LE', 'unsigned', 'Standard', '0', '0.125', '0', '0', '8031.875'; 'SAofContrDeviceforEngCtrl', '40', '8', 'LE', 'unsigned', 'Standard', '0', '1', '0', '0', '255' }
      settings: SourceProductBaseCode=ME,XP,VN  DataFormat=manually specified signals
  Data Store Read1 : DataStoreRead  DataStoreName=OutputNetworkData  DataStoreElements=OutputNetworkData.CCAN.EEC1.ActEngPercentTrq#OutputNetworkData.CCAN.EEC1.ActEngPercentTrqHR#OutputNetworkData.CCAN.EEC1.DrvrsDemandEngPercTrq#OutputNetworkData.CCAN.EEC1.EngDemantPercTrq#OutputNetworkData.CCAN.EEC1.EngStarterMode#OutputNetworkData.CCAN.EEC1.EngTorqMode#OutputNetworkData.CCAN.EEC1.EngineSpeed#OutputNetworkData.CCAN.EEC1.SAofContrDeviceforEngCtrl
  Terminator1 : Terminator
  transmit_message_eec1 : TTlibrary/CAN/transmit_message_name  channel=IO_CAN_CHANNEL_1  id_format=IO_CAN_STD_FRAME  retranslation=off  io_error=on  sample_time=-1
      settings: SourceProductName=TT control 500 series
  wires:
  Data Store Read1/8 -> CANPack_EEC1/8
  Data Store Read1/7 -> CANPack_EEC1/7
  Data Store Read1/6 -> CANPack_EEC1/6
  Data Store Read1/5 -> CANPack_EEC1/5
  Data Store Read1/4 -> CANPack_EEC1/4
  Data Store Read1/3 -> CANPack_EEC1/3
  Data Store Read1/2 -> CANPack_EEC1/2
  Data Store Read1/1 -> CANPack_EEC1/1
  CANPack_EEC1/1 -> transmit_message_eec1/1
  transmit_message_eec1/1 -> Terminator1/1  "error_tx_transmit_message_eec1"

== system VCU_SW/OutputLayer/OutputNetwork/OutputCCAN/SetCCAN50msec/EEC2 ==
  CANPack_EEC2 : canmsglib/CAN Pack  MsgList=(none)  MsgName=EEC2  MsgIDType=Extended (29-bit identifier)  MsgIdentifier=418382842  MsgLength=8  Remote=off  ApplyMinMax=off  BusOutput=on  SignalInfo={ 'AccPedPos1', '8', '8', 'LE', 'unsigned', 'Standard', '0', '0.4', '0', '0', '100'; 'AccPedPos2', '32', '8', 'LE', 'unsigned', 'Standard', '0', '0.4', '0', '0', '100' }
      settings: SourceProductBaseCode=ME,XP,VN  DataFormat=manually specified signals
  Data Store Read1 : DataStoreRead  DataStoreName=OutputNetworkData  DataStoreElements=OutputNetworkData.CCAN.EEC2.AccPedPos1#OutputNetworkData.CCAN.EEC2.AccPedPos2
  Terminator1 : Terminator
  transmit_message_eec2 : TTlibrary/CAN/transmit_message_name  channel=IO_CAN_CHANNEL_1  id_format=IO_CAN_STD_FRAME  retranslation=off  io_error=on  sample_time=-1
      settings: SourceProductName=TT control 500 series
  wires:
  Data Store Read1/2 -> CANPack_EEC2/2
  Data Store Read1/1 -> CANPack_EEC2/1
  CANPack_EEC2/1 -> transmit_message_eec2/1
  transmit_message_eec2/1 -> Terminator1/1  "error_tx_transmit_message_eec2"

== system VCU_SW/OutputLayer/OutputNetwork/OutputDiagCAN + Logger/SetDiagCAN10msec/Simulink Function ==
  getUDSMsg : TriggerPort  TriggerType=function-call  IsSimulinkFunction=on  FunctionName=getUDSMsg  FunctionVisibility=scoped  VariantControl=(inherit)
  MATLAB Function1 : MATLAB Function  TreatAsAtomicUnit=on
  Simulink Function2 : Subsystem  TreatAsAtomicUnit=on
  Simulink Function3 : Subsystem  TreatAsAtomicUnit=on

== system VCU_SW/OutputLayer/OutputNetwork/OutputDiagCAN + Logger/SetDiagCAN10msec1/Simulink Function ==
  getUDSMsg : TriggerPort  TriggerType=function-call  IsSimulinkFunction=on  FunctionName=getUDSMsg  FunctionVisibility=scoped  VariantControl=(inherit)
  MATLAB Function1 : MATLAB Function  TreatAsAtomicUnit=on
  Simulink Function2 : Subsystem  TreatAsAtomicUnit=on
  Simulink Function3 : Subsystem  TreatAsAtomicUnit=on

== system VCU_SW/OutputLayer/OutputNetwork/OutputEngCAN/SetEngCAN50msec/Function-Call Subsystem1 ==
  In1 : Inport
  error_sts : Inport  Port=2
  Enable : EnablePort
  Terminator : Terminator
  Terminator1 : Terminator
  wires:
  In1/1 -> Terminator1/1
  error_sts/1 -> Terminator/1

== system VCU_SW/OutputLayer/OutputNetwork/OutputHydCAN/SetHydCAN100msec/Cabine1stLeftHydCylValve ==
  CANPack_VLVCMD_HYD2 : canmsglib/CAN Pack  MsgList=(none)  MsgName=VLVCMD_HYD2  MsgIDType=Extended (29-bit identifier)  MsgIdentifier=217985530  MsgLength=3  Remote=off  ApplyMinMax=off  BusOutput=on  SignalInfo={ 'FailSafeModeCmdHyd2', '22', '2', 'LE', 'unsigned', 'Standard', '0', '1', '0', '0', '3'; 'PortFlowCmdHyd2', '0', '8', 'LE', 'unsigned', 'Standard', '0', '0.4', '0', '0', '100'; 'ValveStateHyd2', '16', '4', 'LE', 'unsigned', 'Standard', '0', '1', '0', '0', '15' }
      settings: SourceProductBaseCode=ME,XP,VN  DataFormat=manually specified signals
  Data Store Read1 : DataStoreRead  DataStoreName=OutputNetworkData  DataStoreElements=OutputNetworkData.HydCAN.out_CabineTilt_1LeftHydCyl.failSafeModeCmdHyd#OutputNetworkData.HydCAN.out_CabineTilt_1LeftHydCyl.portFlowCmdHyd#OutputNetworkData.HydCAN.out_CabineTilt_1LeftHydCyl.valveStateHyd
  Terminator1 : Terminator
  transmit_message_vlvcmd_hyd2 : TTlibrary/CAN/transmit_message_name  channel=IO_CAN_CHANNEL_0  id_format=IO_CAN_EXT_FRAME  retranslation=off  io_error=on  sample_time=-1
      settings: SourceProductName=TT control 500 series
  wires:
  Data Store Read1/2 -> CANPack_VLVCMD_HYD2/2
  CANPack_VLVCMD_HYD2/1 -> transmit_message_vlvcmd_hyd2/1
  transmit_message_vlvcmd_hyd2/1 -> Terminator1/1  "error_tx_transmit_message_vlvcmd_hyd2"
  Data Store Read1/1 -> CANPack_VLVCMD_HYD2/1
  Data Store Read1/3 -> CANPack_VLVCMD_HYD2/3

== system VCU_SW/OutputLayer/OutputNetwork/OutputHydCAN/SetHydCAN100msec/Cabine2ndRightHydCylValve ==
  CANPack_VLVCMD_HYD3 : canmsglib/CAN Pack  MsgList=(none)  MsgName=VLVCMD_HYD3  MsgIDType=Extended (29-bit identifier)  MsgIdentifier=217985786  MsgLength=3  Remote=off  ApplyMinMax=off  BusOutput=on  SignalInfo={ 'FailSafeModeCmdHyd3', '22', '2', 'LE', 'unsigned', 'Standard', '0', '1', '0', '0', '3'; 'PortFlowCmdHyd3', '0', '8', 'LE', 'unsigned', 'Standard', '0', '0.4', '0', '0', '100'; 'ValveStateHyd3', '16', '4', 'LE', 'unsigned', 'Standard', '0', '1', '0', '0', '15' }
      settings: SourceProductBaseCode=ME,XP,VN  DataFormat=manually specified signals
  Data Store Read1 : DataStoreRead  DataStoreName=OutputNetworkData  DataStoreElements=OutputNetworkData.HydCAN.out_CabineTilt_2RightHydCyl.failSafeModeCmdHyd#OutputNetworkData.HydCAN.out_CabineTilt_2RightHydCyl.portFlowCmdHyd#OutputNetworkData.HydCAN.out_CabineTilt_2RightHydCyl.valveStateHyd
  Terminator1 : Terminator
  transmit_message_vlvcmd_hyd3 : TTlibrary/CAN/transmit_message_name  channel=IO_CAN_CHANNEL_0  id_format=IO_CAN_EXT_FRAME  retranslation=off  io_error=on  sample_time=-1
      settings: SourceProductName=TT control 500 series
  wires:
  Data Store Read1/3 -> CANPack_VLVCMD_HYD3/3
  Data Store Read1/1 -> CANPack_VLVCMD_HYD3/1
  transmit_message_vlvcmd_hyd3/1 -> Terminator1/1  "error_tx_transmit_message_vlvcmd_hyd3"
  CANPack_VLVCMD_HYD3/1 -> transmit_message_vlvcmd_hyd3/1
  Data Store Read1/2 -> CANPack_VLVCMD_HYD3/2

== system VCU_SW/OutputLayer/OutputNetwork/OutputHydCAN/SetHydCAN100msec/CabineTurningValve ==
  CANPack_VLVCMD_HYD1 : canmsglib/CAN Pack  MsgList=(none)  MsgName=VLVCMD_HYD1  MsgIDType=Extended (29-bit identifier)  MsgIdentifier=217985274  MsgLength=3  Remote=off  ApplyMinMax=off  BusOutput=on  SignalInfo={ 'FailSafeModeCmdHyd1', '22', '2', 'LE', 'unsigned', 'Standard', '0', '1', '0', '0', '3'; 'PortFlowCmdHyd1', '0', '8', 'LE', 'unsigned', 'Standard', '0', '0.4', '0', '0', '100'; 'ValveStateHyd1', '16', '4', 'LE', 'unsigned', 'Standard', '0', '1', '0', '0', '15' }
      settings: SourceProductBaseCode=ME,XP,VN  DataFormat=manually specified signals
  Data Store Read1 : DataStoreRead  DataStoreName=OutputNetworkData  DataStoreElements=OutputNetworkData.HydCAN.out_CabineRotationVlv.failSafeModeCmdHyd#OutputNetworkData.HydCAN.out_CabineRotationVlv.portFlowCmdHyd#OutputNetworkData.HydCAN.out_CabineRotationVlv.valveStateHyd
  Terminator1 : Terminator
  transmit_message_vlvcmd_hyd1 : TTlibrary/CAN/transmit_message_name  channel=IO_CAN_CHANNEL_0  id_format=IO_CAN_EXT_FRAME  retranslation=off  io_error=on  sample_time=-1
      settings: SourceProductName=TT control 500 series
  wires:
  Data Store Read1/3 -> CANPack_VLVCMD_HYD1/3
  Data Store Read1/1 -> CANPack_VLVCMD_HYD1/1
  transmit_message_vlvcmd_hyd1/1 -> Terminator1/1  "error_tx_transmit_message_vlvcmd_hyd1"
  CANPack_VLVCMD_HYD1/1 -> transmit_message_vlvcmd_hyd1/1
  Data Store Read1/2 -> CANPack_VLVCMD_HYD1/2

== system VCU_SW/InputLayer/InputInterfaces/AnalogInput/AIProc1000msec/TemperatureValues/calcCurPressSensVal ==
  calcCurPressSens : TriggerPort  TriggerType=function-call  IsSimulinkFunction=on  FunctionName=calcCurPressSens  FunctionVisibility=scoped  VariantControl=(inherit)
  Constant12 : Constant  Value=pTempSensAccVolt
  Constant8 : Constant  Value=pMaxTempSensVoltage
  Constant9 : Constant  Value=pMinTempSensVoltage
  MATLAB Function1 : MATLAB Function  TreatAsAtomicUnit=on
  sensValue : ArgIn  DisableCoverage=on  OutDataTypeStr=uint16  ArgumentName=sensValue
  tempMax : ArgIn  Port=2  OutDataTypeStr=int16  ArgumentName=tempMax
  tempMin : ArgIn  Port=3  OutDataTypeStr=int16  ArgumentName=tempMin
  tempValue : ArgOut  DisableCoverage=on  OutDataTypeStr=int16  ArgumentName=tempValue
  wires:
  Constant8/1 -> MATLAB Function1/1(maxValue)
  sensValue/1 -> MATLAB Function1/3(sensorValue)
  Constant9/1 -> MATLAB Function1/2(minValue)
  tempMin/1 -> MATLAB Function1/5(minTemp)
  tempMax/1 -> MATLAB Function1/6(maxTemp)
  Constant12/1 -> MATLAB Function1/4(accuracyValue)
  MATLAB Function1/1(temperature) -> tempValue/1
